simulink library "AMKMotor"  (R2017b)
settings: Solver=ode45  StartTime=0.0  StopTime=10.0  RelTol=1e-3  EnableMultiTasking=on
undefined symbols (not defined in the file): Motor
libraries: simulink x1
settings Model: Creator=BRIAN  LastModifiedBy=Harjot
settings DataIOCC: LimitDataPoints=on  SaveFormat=Array
settings OptimizationCC: LifeSpan=inf
settings DebuggingCC: SFUnexpectedBacktrackingDiag=warning  SFNoUnconditionalDefaultTransitionDiag=warning  SFExecutionAtInitializationDiag=none
settings HardwareCC: ProdBitPerPointer=32  ProdBitPerSizeT=32  ProdBitPerPtrDiffT=32  ProdLargestAtomicFloat=None  ProdIntDivRoundTo=Undefined  ProdEndianess=Unspecified  ProdWordSize=32  ProdHWDeviceType=32-bit Generic
settings ModelReferenceCC: PropagateSignalLabelsOutOfModel=off
settings CodeAppCC: StateflowObjectComments=on
settings GRTTargetCC: TargetLangStandard=C89/C90 (ANSI)  GeneratePreprocessorConditionals=Disable all
settings ConfigComp: CovMetricSettings=dw  CovHtmlReporting=on  CovSaveCumulativeToWorkspaceVar=on  CovSaveSingleToWorkspaceVar=on  CovExternalEMLEnable=off

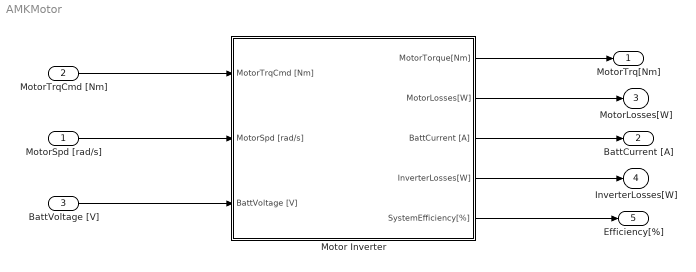
== system AMKMotor ==
  MotorSpd [rad/s] : Inport
  MotorTrqCmd [Nm] : Inport  Port=2
  BattVoltage [V] : Inport  Port=3
  Motor Inverter : Subsystem
  MotorTrq[Nm] : Outport
  BattCurrent [A] : Outport  Port=2
  MotorLosses[W] : Outport  Port=3
  InverterLosses[W] : Outport  Port=4
  Efficiency[%] : Outport  Port=5
  wires:
  MotorTrqCmd [Nm]/1 -> Motor Inverter/1(MotorTrqCmd [Nm])
  MotorSpd [rad/s]/1 -> Motor Inverter/2(MotorSpd [rad/s])
  Motor Inverter/1(MotorTorque[Nm]) -> MotorTrq[Nm]/1
  Motor Inverter/2(MotorLosses[W]) -> MotorLosses[W]/1
  BattVoltage [V]/1 -> Motor Inverter/3(BattVoltage [V])
  Motor Inverter/4(InverterLosses[W]) -> InverterLosses[W]/1
  Motor Inverter/5(SystemEfficiency[%]) -> Efficiency[%]/1
  Motor Inverter/3(BattCurrent [A]) -> BattCurrent [A]/1

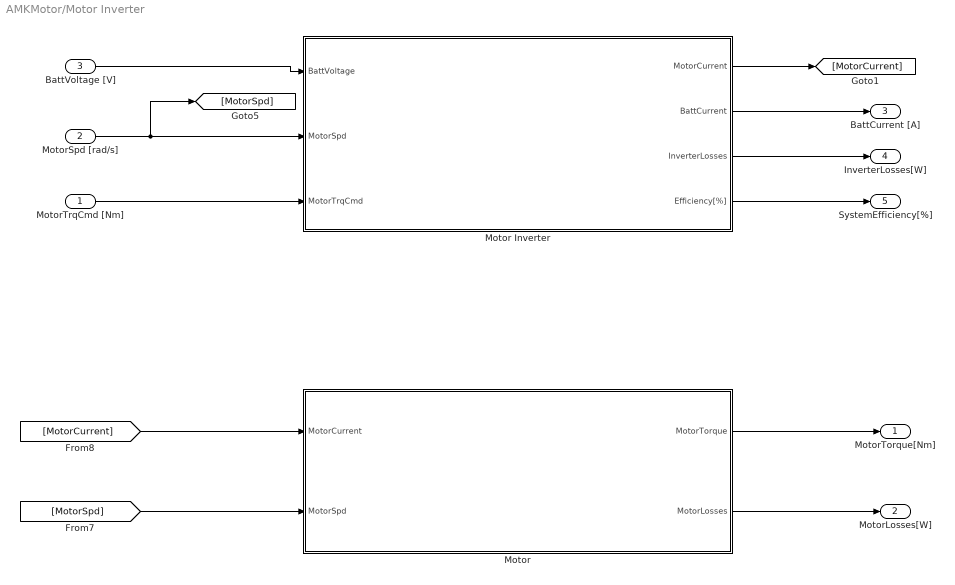
== system AMKMotor/Motor Inverter ==
  MotorTrqCmd [Nm] : Inport
  MotorSpd [rad/s] : Inport  Port=2
  BattVoltage [V] : Inport  Port=3
  Motor : Subsystem
  Motor Inverter : Subsystem
  MotorTorque[Nm] : Outport
  MotorLosses[W] : Outport  Port=2
  BattCurrent [A] : Outport  Port=3
  InverterLosses[W] : Outport  Port=4
  SystemEfficiency[%] : Outport  Port=5
  wires:
  Motor Inverter/4(Efficiency[%]) -> SystemEfficiency[%]/1
  Motor/2(MotorLosses) -> MotorLosses[W]/1
  Motor Inverter/3(InverterLosses) -> InverterLosses[W]/1
  Motor Inverter/1(MotorCurrent) -> [MotorCurrent]
  Motor Inverter/2(BattCurrent) -> BattCurrent [A]/1
  Motor/1(MotorTorque) -> MotorTorque[Nm]/1
  [MotorSpd] -> Motor/2(MotorSpd)
  [MotorCurrent] -> Motor/1(MotorCurrent)
  MotorTrqCmd [Nm]/1 -> Motor Inverter/3(MotorTrqCmd)
  MotorSpd [rad/s]/1 -> Motor Inverter/2(MotorSpd), [MotorSpd]
  BattVoltage [V]/1 -> Motor Inverter/1(BattVoltage)

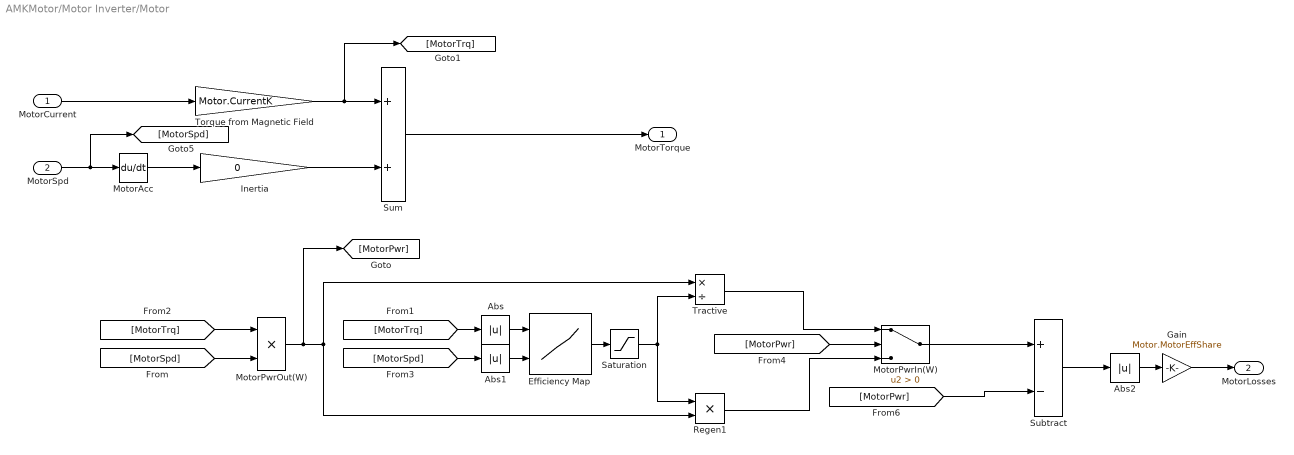
== system AMKMotor/Motor Inverter/Motor ==
  MotorCurrent : Inport
  MotorSpd : Inport  Port=2
  Abs : Abs
  Abs1 : Abs
  Abs2 : Abs
  Efficiency Map : Lookup_n-D  BreakpointsForDimension1=Motor.Efficiency.Trq  BreakpointsForDimension2=Motor.Efficiency.Spd  Table=Motor.Efficiency.Eff  InternalRulePriority=Speed  RndMeth=Simplest  InputSameDT=on
  Gain : Gain  Gain=Motor.MotorEffShare
  Inertia : Gain  Gain=0
  MotorAcc : Derivative
  MotorPwrIn(W) : Switch  Criteria=u2 > Threshold
  MotorPwrOut(W) : Product
  Regen1 : Product
  Saturation : Saturate  UpperLimit=1  LowerLimit=0.01
  Subtract : Sum  Inputs=+-
  Sum : Sum
  Torque from Magnetic Field : Gain  Gain=Motor.CurrentK
  Tractive : Product  Inputs=*/
  MotorTorque : Outport
  MotorLosses : Outport  Port=2
  wires:
  Gain/1 -> MotorLosses/1
  Abs2/1 -> Gain/1
  Subtract/1 -> Abs2/1
  [MotorPwr] -> Subtract/2
  Abs1/1 -> Efficiency Map/2
  Abs/1 -> Efficiency Map/1
  Saturation/1 -> Tractive/2, Regen1/1
  MotorPwrIn(W)/1 -> Subtract/1
  Regen1/1 -> MotorPwrIn(W)/3
  Tractive/1 -> MotorPwrIn(W)/1
  Efficiency Map/1 -> Saturation/1
  MotorPwrOut(W)/1 -> Tractive/1, Regen1/2, [MotorPwr]
  [MotorPwr] -> MotorPwrIn(W)/2
  [MotorSpd] -> Abs1/1
  [MotorTrq] -> MotorPwrOut(W)/1
  [MotorTrq] -> Abs/1
  [MotorSpd] -> MotorPwrOut(W)/2
  MotorAcc/1 -> Inertia/1
  MotorCurrent/1 -> Torque from Magnetic Field/1
  MotorSpd/1 -> MotorAcc/1, [MotorSpd]
  Torque from Magnetic Field/1 -> Sum/1, [MotorTrq]
  Sum/1 -> MotorTorque/1
  Inertia/1 -> Sum/2

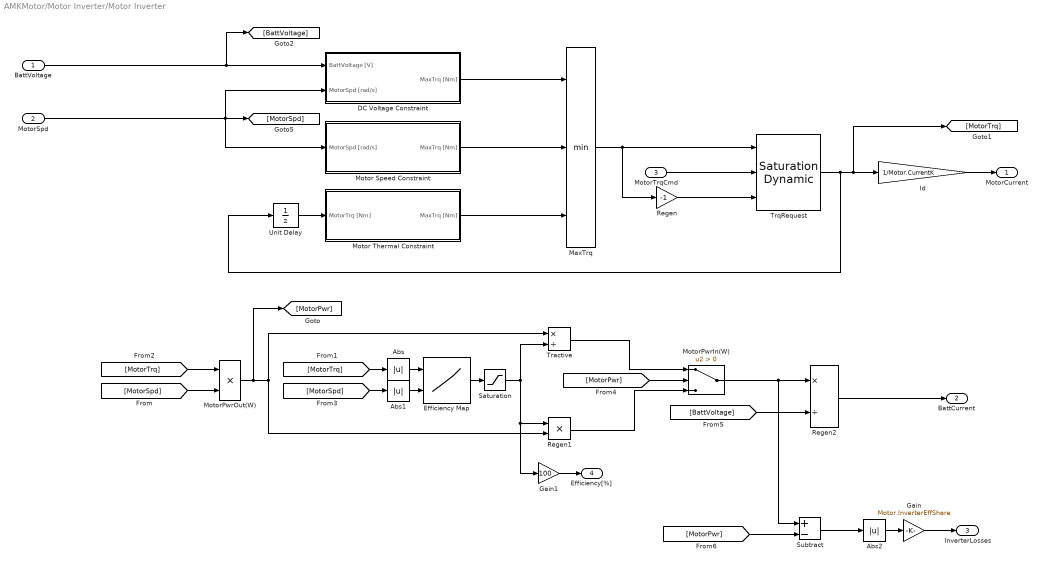
== system AMKMotor/Motor Inverter/Motor Inverter ==
  BattVoltage : Inport
  MotorSpd : Inport  Port=2
  MotorTrqCmd : Inport  Port=3
  Abs : Abs
  Abs1 : Abs
  Abs2 : Abs
  DC Voltage Constraint : Subsystem
  Efficiency Map : Lookup_n-D  BreakpointsForDimension1=Motor.Efficiency.Trq  BreakpointsForDimension2=Motor.Efficiency.Spd  Table=Motor.Efficiency.Eff  InternalRulePriority=Speed  RndMeth=Simplest  InputSameDT=on
  Gain : Gain  Gain=Motor.InverterEffShare
  Gain1 : Gain  Gain=100
  Id : Gain  Gain=1/Motor.CurrentK
  MaxTrq : MinMax  Inputs=3
  Motor Speed Constraint : Subsystem
  Motor Thermal Constraint : Subsystem
  MotorPwrIn(W) : Switch  Criteria=u2 > Threshold
  MotorPwrOut(W) : Product
  Regen : Gain  Gain=-1
  Regen1 : Product
  Regen2 : Product  Inputs=*/
  Saturation : Saturate  UpperLimit=1  LowerLimit=0.01
  Subtract : Sum  Inputs=+-
  Tractive : Product  Inputs=*/
  TrqRequest : simulink/Discontinuities/Saturation Dynamic  OutMin=[]  OutMax=[]  OutDataTypeStr=Inherit: Same as second input  OutDataType=fixdt(1, 16)  OutScaling=2^-10  DoSatur=off
  Unit Delay : UnitDelay  SampleTime=-1
  MotorCurrent : Outport
  BattCurrent : Outport  Port=2
  InverterLosses : Outport  Port=3
  Efficiency[%] : Outport  Port=4
  wires:
  Gain/1 -> InverterLosses/1
  Gain1/1 -> Efficiency[%]/1
  Abs2/1 -> Gain/1
  Subtract/1 -> Abs2/1
  [MotorPwr] -> Subtract/2
  Abs1/1 -> Efficiency Map/2
  Abs/1 -> Efficiency Map/1
  Saturation/1 -> Tractive/2, Regen1/1, Gain1/1
  Regen2/1 -> BattCurrent/1
  [BattVoltage] -> Regen2/2
  MotorPwrIn(W)/1 -> Regen2/1, Subtract/1
  Regen1/1 -> MotorPwrIn(W)/3
  Tractive/1 -> MotorPwrIn(W)/1
  Efficiency Map/1 -> Saturation/1
  MotorPwrOut(W)/1 -> Tractive/1, Regen1/2, [MotorPwr]
  [MotorPwr] -> MotorPwrIn(W)/2
  [MotorSpd] -> Abs1/1
  [MotorTrq] -> MotorPwrOut(W)/1
  [MotorTrq] -> Abs/1
  [MotorSpd] -> MotorPwrOut(W)/2
  Id/1 -> MotorCurrent/1
  Unit Delay/1 -> Motor Thermal Constraint/1(MotorTrq [Nm])
  Motor Thermal Constraint/1(MaxTrq [Nm]) -> MaxTrq/3
  Regen/1 -> TrqRequest/3
  MotorTrqCmd/1 -> TrqRequest/2
  BattVoltage/1 -> DC Voltage Constraint/1(BattVoltage [V]), [BattVoltage]
  DC Voltage Constraint/1(MaxTrq [Nm]) -> MaxTrq/1
  Motor Speed Constraint/1(MaxTrq [Nm]) -> MaxTrq/2
  MotorSpd/1 -> [MotorSpd], Motor Speed Constraint/1(MotorSpd [rad/s]), DC Voltage Constraint/2(MotorSpd [rad/s])
  MaxTrq/1 -> Regen/1, TrqRequest/1
  TrqRequest/1 -> Unit Delay/1, Id/1, [MotorTrq]

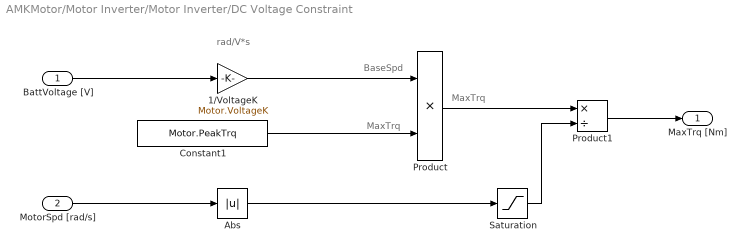
== system AMKMotor/Motor Inverter/Motor Inverter/DC Voltage Constraint ==
  note: MaxTrq
  note: MaxTrq
  note: BaseSpd
  note: rad/V*s
  BattVoltage [V] : Inport
  MotorSpd [rad/s] : Inport  Port=2
  1/VoltageK : Gain  Gain=Motor.VoltageK
  Abs : Abs
  Constant1 : Constant  Value=Motor.PeakTrq
  Product : Product
  Product1 : Product  Inputs=*/
  Saturation : Saturate  UpperLimit=inf  LowerLimit=Motor.MinSpd
  MaxTrq [Nm] : Outport
  wires:
  Saturation/1 -> Product1/2
  Product/1 -> Product1/1
  BattVoltage [V]/1 -> 1/VoltageK/1
  Constant1/1 -> Product/2
  Product1/1 -> MaxTrq [Nm]/1
  MotorSpd [rad/s]/1 -> Abs/1
  1/VoltageK/1 -> Product/1
  Abs/1 -> Saturation/1

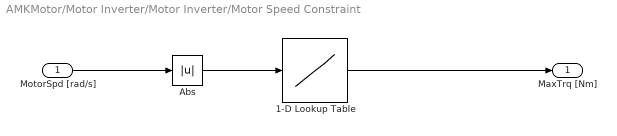
== system AMKMotor/Motor Inverter/Motor Inverter/Motor Speed Constraint ==
  MotorSpd [rad/s] : Inport
  1-D Lookup Table : Lookup_n-D  NumberOfTableDimensions=1  BreakpointsForDimension1=Motor.MaxTrq.Spd  Table=Motor.MaxTrq.Trq  InternalRulePriority=Speed  RndMeth=Simplest  InputSameDT=on
  Abs : Abs
  MaxTrq [Nm] : Outport
  wires:
  MotorSpd [rad/s]/1 -> Abs/1
  1-D Lookup Table/1 -> MaxTrq [Nm]/1
  Abs/1 -> 1-D Lookup Table/1

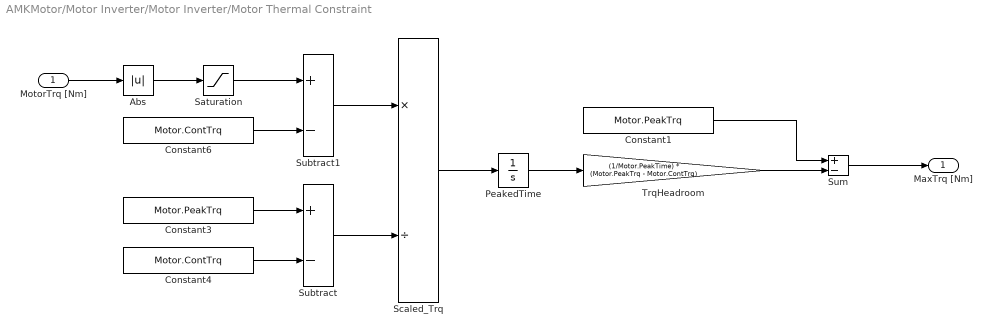
== system AMKMotor/Motor Inverter/Motor Inverter/Motor Thermal Constraint ==
  MotorTrq [Nm] : Inport
  Abs : Abs
  Constant1 : Constant  Value=Motor.PeakTrq
  Constant3 : Constant  Value=Motor.PeakTrq
  Constant4 : Constant  Value=Motor.ContTrq
  Constant6 : Constant  Value=Motor.ContTrq
  PeakedTime : Integrator  LimitOutput=on  LowerSaturationLimit=0
  Saturation : Saturate  UpperLimit=Motor.PeakTrq  LowerLimit=0
  Scaled_Trq : Product  Inputs=*/
  Subtract : Sum  Inputs=+-
  Subtract1 : Sum  Inputs=+-
  Sum : Sum  Inputs=+-
  TrqHeadroom : Gain  Gain=(1/Motor.PeakTime) * (Motor.PeakTrq - Motor.ContTrq)
  MaxTrq [Nm] : Outport
  wires:
  Constant1/1 -> Sum/1
  Sum/1 -> MaxTrq [Nm]/1
  TrqHeadroom/1 -> Sum/2
  Saturation/1 -> Subtract1/1
  PeakedTime/1 -> TrqHeadroom/1
  Abs/1 -> Saturation/1
  Subtract1/1 -> Scaled_Trq/1
  Subtract/1 -> Scaled_Trq/2
  Scaled_Trq/1 -> PeakedTime/1
  Constant6/1 -> Subtract1/2
  Constant3/1 -> Subtract/1
  Constant4/1 -> Subtract/2
  MotorTrq [Nm]/1 -> Abs/1
